simulink model "clik_phi_inverse"  (R2022b)
settings: Solver=ode1  StartTime=0.0  StopTime=4  FixedStep=0.001  RelTol=1e-3
values from neighbouring files (symbols this model uses):
  q0 = [-0.927293431585 -1.28700579042 0.7 2.21429922201]    [matlab.mat]
  Tc = 0.001    [matlab.mat]
undefined symbols (not defined in the file or in its folder): DiscIntNeverNeededParam
settings Model: Creator=Xp  LastModifiedBy=shubham
settings SolverCC: AlgebraicLoopSolver=TrustRegion
settings DataIOCC: LimitDataPoints=on  SaveFormat=Array  SignalLoggingSaveFormat=ModelDataLogs  ReturnWorkspaceOutputs=off
settings OptimizationCC: ExpressionDepthLimit=2147483647  InitFltsAndDblsToZero=on  LifeSpan=inf
settings DebuggingCC: SaveWithParameterizedLinksMsg=none  UnderspecifiedInitializationDetection=Classic  MergeDetectMultiDrivingBlocksExec=none  SolverPrmCheckMsg=warning  MultiTaskDSMMsg=warning  MultiTaskCondExecSysMsg=none  FcnCallInpInsideContextMsg=warning  UnconnectedInputMsg=warning  UnconnectedOutputMsg=warning  UnconnectedLineMsg=warning  StateNameClashWarn=warning  SFUnexpectedBacktrackingDiag=warning  SFNoUnconditionalDefaultTransitionDiag=warning  SFExecutionAtInitializationDiag=none  SFMachineParentedDataDiag=warning  ArithmeticOperatorsInVariantConditions=warning
settings HardwareCC: ProdBitPerPointer=32  ProdBitPerSizeT=32  ProdBitPerPtrDiffT=32  ProdLargestAtomicFloat=None  ProdIntDivRoundTo=Undefined  ProdEndianess=Unspecified  ProdWordSize=32  ProdHWDeviceType=32-bit Generic
settings ModelReferenceCC: EnableRefExpFcnMdlSchedulingChecks=on  PropagateSignalLabelsOutOfModel=off
settings SFSimCC: CustomCodeUndefinedFunction=UseInterfaceOnly
settings RTWCC: DLArmComputeVersion=19.05
settings CodeAppCC: StateflowObjectComments=on
settings GRTTargetCC: TargetLangStandard=C89/C90 (ANSI)  CombineOutputUpdateFcns=off  GRTInterface=on
settings ConfigComp: CovMetricSettings=dw  CovSaveCumulativeToWorkspaceVar=on  CovSaveSingleToWorkspaceVar=on

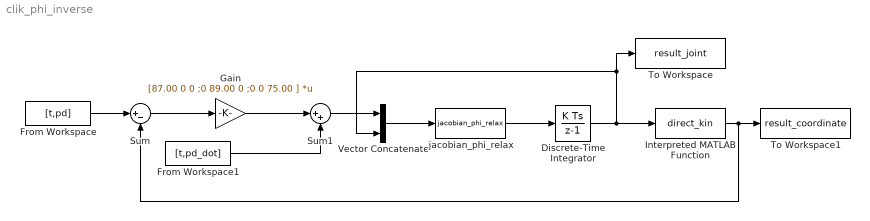
== system clik_phi_inverse ==
  Discrete-Time Integrator : DiscreteIntegrator  InitialCondition=q0  SampleTime=Tc  ICPrevOutput=DiscIntNeverNeededParam  ICPrevScaledInput=DiscIntNeverNeededParam
  From Workspace : FromWorkspace  VariableName=[t,pd]
  From Workspace1 : FromWorkspace  VariableName=[t,pd_dot]  SampleTime=Tc
  Gain : Gain  Gain=[87.00 0 0 ;0 89.00 0 ;0 0 75.00 ]  Multiplication=Matrix(K*u)
  Interpreted MATLAB Function : MATLABFcn  MATLABFcn=direct_kin  OutputDimensions=3  OutputSignalType=real
  Sum : Sum  Inputs=|+-
  Sum1 : Sum  Inputs=|++
  To Workspace : ToWorkspace  VariableName=result_joint  SampleTime=-1
  To Workspace1 : ToWorkspace  VariableName=result_coordinate  SampleTime=-1
  Vector Concatenate : Concatenate
  jacobian_phi_relax : MATLABFcn  MATLABFcn=jacobian_phi_relax
  wires:
  From Workspace/1 -> Sum/1
  Sum/1 -> Gain/1
  Gain/1 -> Sum1/1
  jacobian_phi_relax/1 -> Discrete-Time Integrator/1
  Discrete-Time Integrator/1 -> Interpreted MATLAB Function/1, To Workspace/1, Vector Concatenate/2
  Interpreted MATLAB Function/1 -> To Workspace1/1, Sum/2
  From Workspace1/1 -> Sum1/2
  Sum1/1 -> Vector Concatenate/1
  Vector Concatenate/1 -> jacobian_phi_relax/1
